simulink model "Pole_placement_and_Tracking_control"  (R2023b)
settings: Solver=VariableStepAuto  StartTime=0.0  StopTime=200.0  RelTol=1e-3
undefined symbols (not defined in the file or in its folder): A_uns, B_uns, K_pp, x1_bar_uns, x3_bar_uns
libraries: simulink_extras x4
settings Model: Creator=Mark  LastModifiedBy=Mark

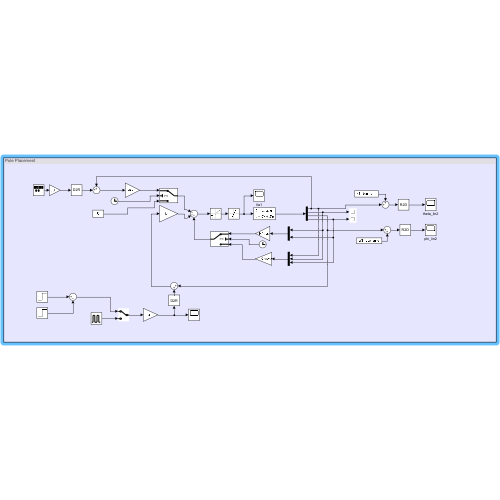
[thumbnail: Simulink's stored preview of the top-level diagram]
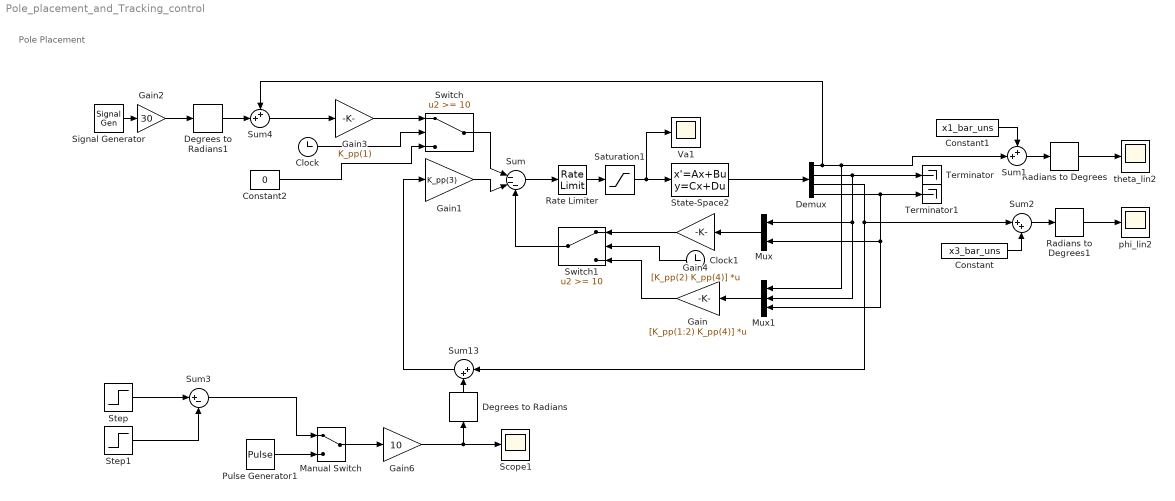
== system Pole_placement_and_Tracking_control ==
  note: Pole Placement
  Clock : Clock
  Clock1 : Clock
  Constant : Constant  Value=x3_bar_uns
  Constant1 : Constant  Value=x1_bar_uns
  Constant2 : Constant  Value=0
  Degrees to Radians : simulink_extras/Transformations/Degrees to Radians
  Degrees to Radians1 : simulink_extras/Transformations/Degrees to Radians
  Demux : Demux
  Gain : Gain  Gain=[K_pp(1:2) K_pp(4)]  Multiplication=Matrix(K*u) (u vector)
  Gain1 : Gain  Gain=K_pp(3)
  Gain2 : Gain  Gain=30
  Gain3 : Gain  Gain=K_pp(1)
  Gain4 : Gain  Gain=[K_pp(2) K_pp(4)]  Multiplication=Matrix(K*u) (u vector)
  Gain6 : Gain  Gain=10
  Manual Switch : ManualSwitch
  Mux : Mux  Inputs=2
  Mux1 : Mux  Inputs=3
  Pulse Generator1 : DiscretePulseGenerator  PulseType=Time based  Period=10000  PulseWidth=0.005  PhaseDelay=30
  Radians to Degrees : simulink_extras/Transformations/Radians to Degrees
  Radians to Degrees1 : simulink_extras/Transformations/Radians to Degrees
  Rate Limiter : RateLimiter  RisingSlewLimit=inf  FallingSlewLimit=-inf  SampleTimeMode=inherited
  Saturation1 : Saturate  UpperLimit=10  LowerLimit=-10
  Scope1 : Scope
  Signal Generator : SignalGenerator  Frequency=0.05
  State-Space2 : StateSpace  A=A_uns  B=B_uns  C=eye(4)  D=zeros(4,1)  InitialCondition=[0 0 0 0]  ParameterTunability=Optimized
  Step : Step  Time=35  SampleTime=0
  Step1 : Step  Time=35.005  SampleTime=0
  Sum : Sum  Inputs=|---
  Sum1 : Sum  Inputs=++|
  Sum13 : Sum  Inputs=|++
  Sum2 : Sum  Inputs=|++
  Sum3 : Sum  Inputs=|+-
  Sum4 : Sum  Inputs=++|
  Switch : Switch  Threshold=10  SaturateOnIntegerOverflow=off  InputSameDT=off
  Switch1 : Switch  Threshold=10  SaturateOnIntegerOverflow=off  InputSameDT=off
  Terminator : Terminator
  Terminator1 : Terminator
  Va1 : Scope
  phi_lin2 : Scope
  theta_lin2 : Scope
  wires:
  Sum13/1 -> Gain1/1
  Mux1/1 -> Gain/1
  Sum2/1 -> Radians to Degrees1/1
  Step/1 -> Sum3/1
  Demux/3 -> Sum13/1, Sum2/1
  Sum3/1 -> Manual Switch/1
  Constant1/1 -> Sum1/1
  Step1/1 -> Sum3/2
  Sum1/1 -> Radians to Degrees/1
  Rate Limiter/1 -> Saturation1/1
  Degrees to Radians/1 -> Sum13/2
  Demux/2 -> Mux/1, Mux1/2, Terminator/1
  Demux/4 -> Terminator1/1, Mux/2, Mux1/3
  Radians to Degrees1/1 -> phi_lin2/1
  Gain1/1 -> Sum/2
  Gain/1 -> Switch1/3
  Constant/1 -> Sum2/2
  Manual Switch/1 -> Gain6/1
  Radians to Degrees/1 -> theta_lin2/1
  Sum/1 -> Rate Limiter/1
  Gain6/1 -> Scope1/1, Degrees to Radians/1
  State-Space2/1 -> Demux/1
  Pulse Generator1/1 -> Manual Switch/2
  Saturation1/1 -> Va1/1, State-Space2/1
  Demux/1 -> Sum4/1, Mux1/1, Sum1/2
  Signal Generator/1 -> Gain2/1
  Sum4/1 -> Gain3/1
  Gain2/1 -> Degrees to Radians1/1
  Gain3/1 -> Switch/1
  Switch/1 -> Sum/1
  Clock/1 -> Switch/2
  Constant2/1 -> Switch/3
  Degrees to Radians1/1 -> Sum4/2
  Mux/1 -> Gain4/1
  Gain4/1 -> Switch1/1
  Clock1/1 -> Switch1/2
  Switch1/1 -> Sum/3
